simulink model "s_aero_2dof_pid_control"  (R2014a)
settings: Solver=ode1  StartTime=0.0  StopTime=30  FixedStep=0.002  RelTol=1e-3
values from neighbouring files (symbols this model uses):
  kd_y = (2*tau*zeta*wn-1)/K    [quanser_aero_pd_design.m]    (also in quanser_aero_pd_design_Ksp.m = (2*Jy*zeta*wn-Dy)/Kyy)
  kp_p = tau*wn^2/K    [quanser_aero_pd_design.m]    (also in quanser_aero_pd_design_Ksp.m = (Jp*wn^2-Ksp)/Kpp)
  kp_y = tau*wn^2/K    [quanser_aero_pd_design.m]    (also in quanser_aero_pd_design_Ksp.m = Jy*wn^2/Kyy)
undefined symbols (not defined in the file or in its folder): Dp, Dy, Jp, Jy, Kpp, Kpy, Ksp, Kyp, Kyy
libraries: simulink_extras x4, quarc_library x3
settings Model: ExtModeTrigDuration=5000  Creator=MLevis  LastModifiedBy=MLevis
settings SolverCC: PositivePriorityOrder=on
settings DebuggingCC: MergeDetectMultiDrivingBlocksExec=error
settings RTWCC: SystemTargetFile=quarc_win64.tlc  TemplateMakefile=quarc_default_tmf  Description=QUARC Win64 Target  ProcessScript=quarc_win64_make_rtw_hook
settings GRTTargetCC: ParMdlRefBuildCompliant=off  CompOptLevelCompliant=off  CombineOutputUpdateFcns=off  MatFileLogging=off  CPPClassGenCompliant=off  GRTInterface=on  ExtMode=on  ExtModeMexFile=quarc_comm

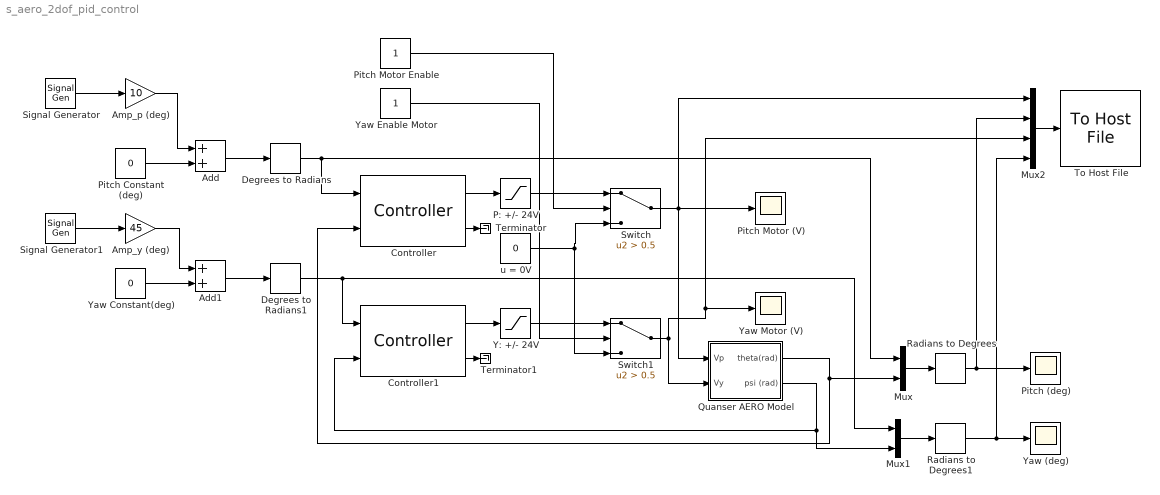
== system s_aero_2dof_pid_control ==
  Add : Sum
  Add1 : Sum
  Amp_p (deg) : Gain  Gain=10
  Amp_y (deg) : Gain  Gain=45
  Controller : quarc_library/Continuous/Controller  ctrl_type=Proportional-Integral-Velocity (PIV)  param_src=Specify via dialog  Kp=kp_p  Ki=0  Kd=0  Kv=kd_p  Ka=0  Wn=100
  Controller1 : quarc_library/Continuous/Controller  ctrl_type=Proportional-Integral-Velocity (PIV)  param_src=Specify via dialog  Kp=kp_y  Ki=0  Kd=kd_y  Kv=kd_y  Ka=0  Wn=100
  Degrees to Radians : simulink_extras/Transformations/Degrees to Radians
  Degrees to Radians1 : simulink_extras/Transformations/Degrees to Radians
  Mux : Mux  Inputs=2
  Mux1 : Mux  Inputs=2
  Mux2 : Mux
  P: +/- 24V : Saturate  UpperLimit=24  LowerLimit=-24
  Pitch (deg) : Scope
      settings: TimeRange=30  YMin=-45  YMax=45  SaveName=ScopeData3  MaxDataPoints=15000
  Pitch Constant (deg) : Constant  Value=0
  Pitch Motor (V) : Scope
      settings: TimeRange=30  YMin=-25  YMax=25  SaveName=ScopeData2  MaxDataPoints=15000
  Pitch Motor Enable : Constant
  Quanser AERO Model : Subsystem
  Radians to Degrees : simulink_extras/Transformations/Radians to Degrees
  Radians to Degrees1 : simulink_extras/Transformations/Radians to Degrees
  Signal Generator : SignalGenerator  WaveForm=square  Frequency=0.1
  Signal Generator1 : SignalGenerator  WaveForm=square  Frequency=0.04
  Switch : Switch  Criteria=u2 > Threshold  Threshold=0.5
  Switch1 : Switch  Criteria=u2 > Threshold  Threshold=0.5
  Terminator : Terminator
  Terminator1 : Terminator
  To Host File : quarc_library/Sinks/To Host/To Host File  file_name=aero_pid_rsp_sim.mat  variable_name=pid_rsp_sim  decimation=1  sample_time=-1  file_format=MAT-file v.4  options=No header or footer  append=off  final_file_name=aero_pid_rsp_sim.mat
  Y: +/- 24V : Saturate  UpperLimit=24  LowerLimit=-24
  Yaw (deg) : Scope
      settings: TimeRange=30  YMin=-120  YMax=120  SaveName=ScopeData4  MaxDataPoints=15000
  Yaw Constant(deg) : Constant  Value=0
  Yaw Enable Motor : Constant
  Yaw Motor (V) : Scope
      settings: TimeRange=30  YMin=-25  YMax=25  SaveName=ScopeData5  MaxDataPoints=15000
  u = 0V : Constant  Value=0
  wires:
  Controller/1 -> P: +/- 24V/1
  Degrees to Radians/1 -> Controller/1, Mux/1
  Controller1/1 -> Y: +/- 24V/1
  Degrees to Radians1/1 -> Controller1/1, Mux1/1
  Controller/2 -> Terminator/1
  Controller1/2 -> Terminator1/1
  Pitch Constant (deg)/1 -> Add/2
  Yaw Constant(deg)/1 -> Add1/2
  Amp_p (deg)/1 -> Add/1
  Amp_y (deg)/1 -> Add1/1
  Pitch Motor Enable/1 -> Switch/2
  Yaw Enable Motor/1 -> Switch1/2
  Radians to Degrees/1 -> Mux2/2, Pitch (deg)/1
  Radians to Degrees1/1 -> Mux2/4, Yaw (deg)/1
  Y: +/- 24V/1 -> Switch1/1
  P: +/- 24V/1 -> Switch/1
  u = 0V/1 -> Switch/3, Switch1/3
  Quanser AERO Model/2(psi (rad)) -> Mux1/2, Controller1/2
  Quanser AERO Model/1(theta(rad)) -> Controller/2, Mux/2
  Mux/1 -> Radians to Degrees/1
  Mux1/1 -> Radians to Degrees1/1
  Switch/1 -> Mux2/1, Quanser AERO Model/1(Vp), Pitch Motor (V)/1
  Switch1/1 -> Quanser AERO Model/2(Vy), Mux2/3, Yaw Motor (V)/1
  Mux2/1 -> To Host File/1
  Add1/1 -> Degrees to Radians1/1
  Add/1 -> Degrees to Radians/1
  Signal Generator/1 -> Amp_p (deg)/1
  Signal Generator1/1 -> Amp_y (deg)/1

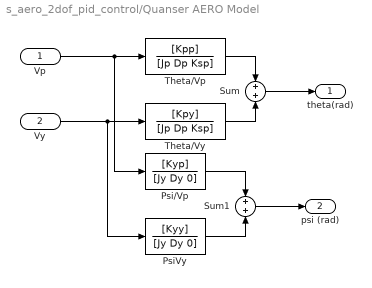
== system s_aero_2dof_pid_control/Quanser AERO Model ==
  Vp : Inport
  Vy : Inport  Port=2
  Psi/Vp : TransferFcn  Numerator=[Kyp]  Denominator=[Jy Dy 0]
  PsiVy : TransferFcn  Numerator=[Kyy]  Denominator=[Jy Dy 0]
  Sum : Sum
  Sum1 : Sum
  Theta/Vp : TransferFcn  Numerator=[Kpp]  Denominator=[Jp Dp Ksp]
  Theta/Vy : TransferFcn  Numerator=[Kpy]  Denominator=[Jp Dp Ksp]
  theta(rad) : Outport
  psi (rad) : Outport  Port=2
  wires:
  Sum/1 -> theta(rad)/1
  Theta/Vp/1 -> Sum/1
  Psi/Vp/1 -> Sum1/1
  PsiVy/1 -> Sum1/2
  Theta/Vy/1 -> Sum/2
  Vp/1 -> Psi/Vp/1, Theta/Vp/1
  Vy/1 -> PsiVy/1, Theta/Vy/1
  Sum1/1 -> psi (rad)/1
